simulink model "BOOST_CONVERTER"  (R2022b)
settings: Solver=ode4  StartTime=0.0  StopTime=1  RelTol=1e-3
libraries: spsVoltageMeasurementLib x5, spsCurrentMeasurementLib x4, spsSeriesRLCBranchLib x3, spsDCVoltageSourceLib x1, spsDiodeLib x1, spsMosfetLib x1, spspowerguiLib x1
settings Model: Creator=Vishnu Vardhan  LastModifiedBy=PC
settings DebuggingCC: UnconnectedInputMsg=warning  UnconnectedOutputMsg=warning  UnconnectedLineMsg=warning
settings ModelReferenceCC: EnableRefExpFcnMdlSchedulingChecks=on
settings RTWCC: DLArmComputeVersion=19.05

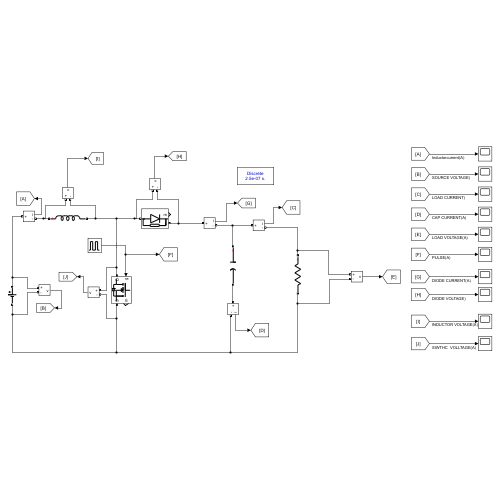
[thumbnail: Simulink's stored preview of the top-level diagram]
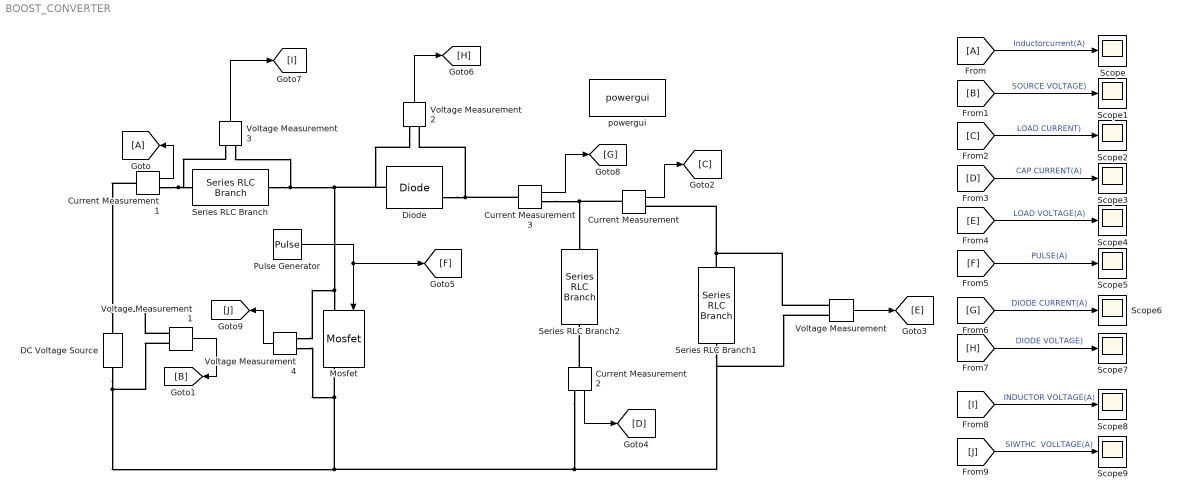
== system BOOST_CONVERTER ==
  Current Measurement{,1..3} (4 alike) : spsCurrentMeasurementLib/Current Measurement  PhasorSimulation=off  OutputType=Complex  PSBequivalent=0
  DC Voltage Source : spsDCVoltageSourceLib/DC Voltage Source  Amplitude=24  Measurements=None
  Diode : spsDiodeLib/Diode  Ron=0.00001  Lon=0  Vf=0.00008  IC=0  UseSnubber=0  Rs=500  Cs=250e-9  Measurements=on
  From : From
  Goto : Goto
  Mosfet : spsMosfetLib/Mosfet  Ron=0.1  Lon=0  Rd=0.01  Vfd=0  IC=0  Rs=1e5  Cs=inf  Measurements=on
  Pulse Generator : DiscretePulseGenerator  PulseType=Time based  Period=1/40000  PulseWidth=0.5*100
  Scope{,1..9} (10 alike) : Scope
  Series RLC Branch : spsSeriesRLCBranchLib/Series RLC Branch  LConnTagsString=__new0  RConnTagsString=__new0  BranchType=L  Resistance=1  Inductance=0.375e-3  SetiL0=off  InitialCurrent=0  Capacitance=1e-6  Setx0=off  InitialVoltage=0  Measurements=None
  Series RLC Branch1 : spsSeriesRLCBranchLib/Series RLC Branch  LConnTagsString=__new0  RConnTagsString=__new0  BranchType=R  Resistance=23.04  Inductance=1e-3  SetiL0=off  InitialCurrent=0  Capacitance=1e-6  Setx0=off  InitialVoltage=0  Measurements=None
  Series RLC Branch2 : spsSeriesRLCBranchLib/Series RLC Branch  LConnTagsString=__new0  RConnTagsString=__new0  BranchType=C  Resistance=1  Inductance=1e-3  SetiL0=off  InitialCurrent=0  Capacitance=5.20825e-3  Setx0=off  InitialVoltage=0  Measurements=None
  Voltage Measurement{,1..4} (5 alike) : spsVoltageMeasurementLib/Voltage Measurement  PhasorSimulation=off  OutputType=Complex  PSBequivalent=0
  powergui : spspowerguiLib/powergui  Priority=1  SimulationMode=Discrete  SampleTime=25e-8  frequency=60  Iterations=50  frequencyindice=0  Pbase=100e6  ErrMax=1e-4  UnitsV=kV  UnitsW=MW  buscounter=0  FunctionMessages=off  echomessages=off  EnableUseOfTLC=off  CurrentSourceSwitches=off  DisableSnubberDevices=off  DisableRonSwitches=off  DisableVfSwitches=off  DisplayEquations=off  AutomaticDiscreteSolvers=off  SolverType=Tustin/Backward Euler (TBE)  Interpol=off  ExternalGateDelay=off  methode=off  Ts=100  x0status=blocks  SPID=on  SwTol=0  HookPort=off  NonlinearTolerance=1e-4  nMaxIteration=100  ContinueOnMaxIteration=off  RestoreLinks=warning  ResistiveCurrentMeasurement=off  Frange=[0:2:500]  Ylog=off  Xlog=on  ShowGrid=off  save=off  variable=ZData  structure=0  ZoomFFT=off  StartTime=0.0  cycles=1  DisplayStyle=1  fundamental=60  FreqAxis=off  MaxFrequency=1000  frequencyindicesteady=1  RmsSteady=1  display=off
  wires:
  Pulse Generator/1 -> [F], Mosfet/1
  Current Measurement1/1 -> Goto/1
  Voltage Measurement1/1 -> [B]
  Current Measurement/1 -> [C]
  Voltage Measurement/1 -> [E]
  Current Measurement2/1 -> [D]
  Voltage Measurement2/1 -> [H]
  Voltage Measurement3/1 -> [I]
  Current Measurement3/1 -> [G]
  Voltage Measurement4/1 -> [J]
  From/1 -> Scope/1  "Inductorcurrent(A)"
  [J] -> Scope9/1  "SIWTHC  VOLLTAGE(A)"
  [I] -> Scope8/1  "INDUCTOR VOLTAGE(A)"
  [H] -> Scope7/1  "DIODE VOLTAGE)"
  [G] -> Scope6/1  "DIODE CURRENT(A)"
  [F] -> Scope5/1  "PULSE(A)"
  [E] -> Scope4/1  "LOAD VOLTAGE(A)"
  [D] -> Scope3/1  "CAP CURRENT(A)"
  [C] -> Scope2/1  "LOAD CURRENT)"
  [B] -> Scope1/1  "SOURCE VOLTAGE)"
  connections:
  Series RLC Branch/RConn1 -- Voltage Measurement3/LConn2 -- Voltage Measurement2/LConn1 -- Diode/LConn1 -- Voltage Measurement4/LConn1 -- Mosfet/LConn1
  DC Voltage Source/LConn1 -- Current Measurement2/RConn1 -- Voltage Measurement/LConn2 -- Series RLC Branch1/RConn1 -- Voltage Measurement4/LConn2 -- Mosfet/RConn1 -- Voltage Measurement1/LConn2
  Current Measurement/LConn1 -- Current Measurement3/RConn1 -- Series RLC Branch2/LConn1
  Series RLC Branch1/LConn1 -- Current Measurement/RConn1 -- Voltage Measurement/LConn1
  Current Measurement1/RConn1 -- Voltage Measurement3/LConn1 -- Series RLC Branch/LConn1
  Current Measurement1/LConn1 -- Voltage Measurement1/LConn1 -- DC Voltage Source/RConn1
  Current Measurement2/LConn1 -- Series RLC Branch2/RConn1
  Diode/RConn1 -- Current Measurement3/LConn1 -- Voltage Measurement2/LConn2
